simulink model "Exp10_2"  (R2018b)
settings: Solver=VariableStepAuto  StartTime=0.0  StopTime=100  RelTol=1e-3
libraries: fuzblock x1
settings Model: Creator=Dear Fatemeh  LastModifiedBy=Dear Fatemeh

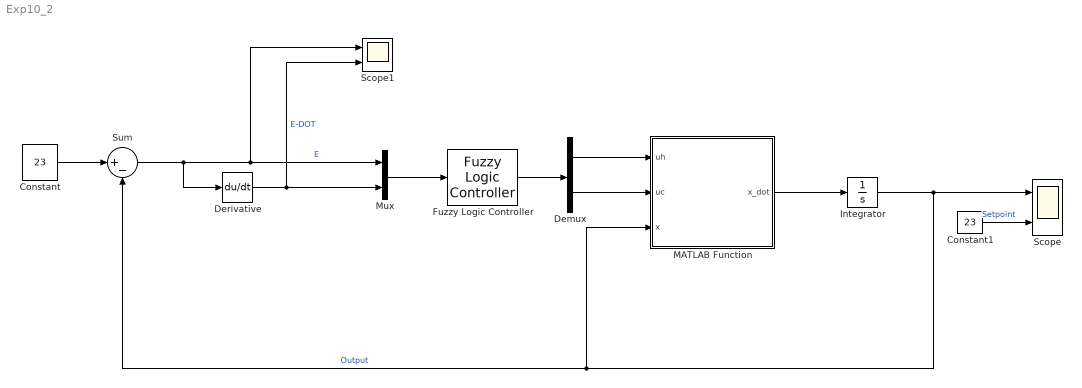
== system Exp10_2 ==
  Constant : Constant  Value=23
  Constant1 : Constant  Value=23
  Demux : Demux  Outputs=2
  Derivative : Derivative
  Fuzzy Logic Controller : fuzblock/Fuzzy Logic  Controller  FIS=Fuzzy_controller2  OutputSampleNumber=101  DataType=double  FuzzifiedInputs=off  RuleFiringStrengths=off  RuleOutputs=off  AggregatedOutputs=off  SimulateUsing=Interpreted execution  OutOfRangeInputValueMessage=warning  NoRuleFiredMessage=warning  EmptyOutputFuzzySetMessage=warning
  Integrator : Integrator  InitialCondition=26
  MATLAB Function : MATLAB Function  TreatAsAtomicUnit=on
  Mux : Mux  Inputs=2
  Scope : Scope  NumInputPorts=2
  Scope1 : Scope  NumInputPorts=2
  Sum : Sum  Inputs=|+-
  wires:
  MATLAB Function/1(x_dot) -> Integrator/1
  Integrator/1 -> Scope/1, Sum/2, MATLAB Function/3(x)  "Output"
  Constant/1 -> Sum/1
  Fuzzy Logic Controller/1 -> Demux/1
  Sum/1 -> Derivative/1, Scope1/1, Mux/1  "E"
  Derivative/1 -> Mux/2, Scope1/2  "E-DOT"
  Constant1/1 -> Scope/2  "Setpoint"
  Demux/1 -> MATLAB Function/1(uh)
  Demux/2 -> MATLAB Function/2(uc)
  Mux/1 -> Fuzzy Logic Controller/1

== matlab function Exp10_2/MATLAB Function ==
  data: uh input; uc input; x input; x_dot output
function x_dot = fcn(uh,uc,x)

x_dot = -0.1*(x-20) + uh - uc;
